simulink model "SAMPLING_SIM"  (R2024a)
settings: Solver=VariableStepAuto  StartTime=0.0  StopTime=10.0  RelTol=1e-3
libraries: dspfdesign x1
settings Model: Creator=adity  LastModifiedBy=adity

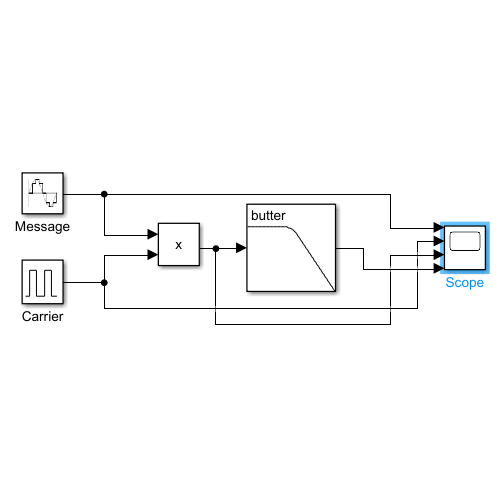
[thumbnail: Simulink's stored preview of the top-level diagram]
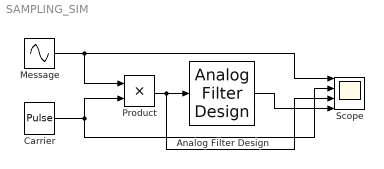
== system SAMPLING_SIM ==
  Analog Filter Design : dspfdesign/Analog Filter Design  method=Butterworth  filttype=Lowpass  N=4  Wlo=30  Whi=80  Rp=2  Rs=40
  Carrier : DiscretePulseGenerator  PulseType=Time based  Period=0.02  PulseWidth=10
  Message : Sin  Frequency=2*pi*1  SampleTime=1/1000
  Product : Product
  Scope : Scope  NumInputPorts=4
  wires:
  Message/1 -> Scope/1, Product/1
  Product/1 -> Scope/3, Analog Filter Design/1
  Carrier/1 -> Scope/2, Product/2
  Analog Filter Design/1 -> Scope/4
